simulink model "test_mambo_close_loop"  (R2022b)
settings: Solver=VariableStepAuto  StartTime=0.0  StopTime=20  RelTol=1e-3
values from neighbouring files (symbols this model uses):
  A_angles = sysd_angles.den    [parrot_mambo_main.m]
  Ad = MLD.A    [parrot_mambo_main.m]
  angle_sat = 0.22    [parrot_mambo_main.m]
  B_angles = sysd_angles.num    [parrot_mambo_main.m]
  Bd = MLD.B    [parrot_mambo_main.m]
  Cd = MLD.C    [parrot_mambo_main.m]
  Dd = MLD.D    [parrot_mambo_main.m]
  delay = 0.08    [parrot_mambo_main.m]
  GLOBAL_PARAMETERS = [Ts m g Kv]    [parrot_mambo_main.m]
  K_gain = dlqr(Ad, Bd, Q_gain_lin, R_gain_lin)    [parrot_mambo_main.m]
  K_gain_lin = lqr(A, B, Q_gain_lin, R_gain_lin)    [parrot_mambo_main.m]
  Ts = 0.01    [parrot_mambo_main.m]
settings Model: Creator=phatdo  LastModifiedBy=phatdo

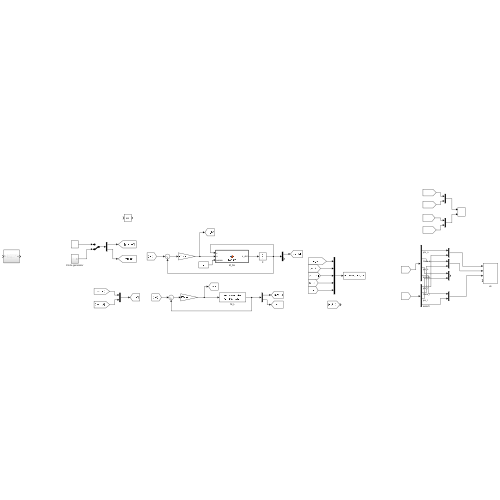
[thumbnail: Simulink's stored preview of the top-level diagram]
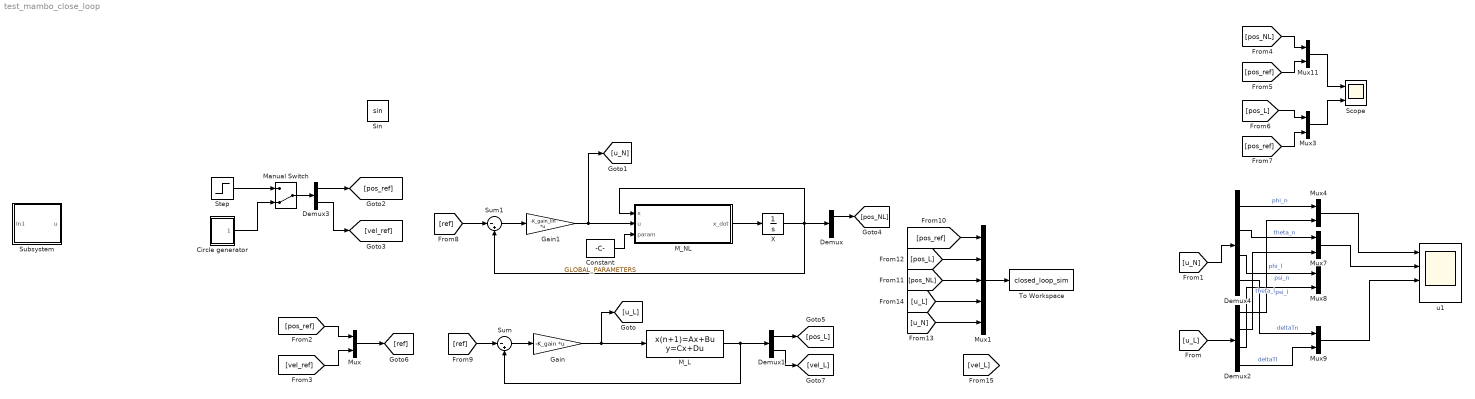
== system test_mambo_close_loop ==
  Circle generator : Subsystem
  Constant : Constant  Value=GLOBAL_PARAMETERS
  Demux : Demux  Outputs=2
  Demux1 : Demux  Outputs=2
  Demux2 : Demux
  Demux3 : Demux  Outputs=2
  Demux4 : Demux
  Gain : Gain  Gain=-K_gain  Multiplication=Matrix(K*u) (u vector)
  Gain1 : Gain  Gain=-K_gain_lin  Multiplication=Matrix(K*u) (u vector)
  M_L : DiscreteStateSpace  A=Ad  B=Bd  C=Cd  D=Dd  SampleTime=-1
  M_NL : MATLAB Function  TreatAsAtomicUnit=on
  Manual Switch : ManualSwitch  CurrentSetting=0
  Mux{,3..4,7..9,11} (7 alike) : Mux  Inputs=2
  Mux1 : Mux  Inputs=5
  Scope : Scope  NumInputPorts=2
  Sin : Trigonometry
  Step : Step  After=[1.5 1.8 2 0 0 0]  SampleTime=Ts
  Subsystem : Subsystem
  Sum : Sum  Inputs=|-+
  Sum1 : Sum  Inputs=|-+
  To Workspace : ToWorkspace  VariableName=closed_loop_sim  SaveFormat=Timeseries  SampleTime=-1
  X : Integrator
  u1 : Scope  NumInputPorts=4
  wires:
  M_L/1 -> Demux1/1, Sum/2
  Sum/1 -> Gain/1
  Gain/1 -> M_L/1, [u_L]
  M_NL/1(x_dot) -> X/1
  Sum1/1 -> Gain1/1
  X/1 -> M_NL/1(x), Demux/1, Sum1/2
  Demux4/1 -> Mux4/1  "phi_n"
  Demux2/1 -> Mux4/2  "phi_l"
  Demux4/2 -> Mux7/1  "theta_n"
  Demux2/2 -> Mux7/2  "theta_l"
  Mux4/1 -> u1/1
  Mux7/1 -> u1/2
  Demux4/3 -> Mux8/1  "psi_n"
  Demux2/3 -> Mux8/2  "psi_l"
  Demux4/4 -> Mux9/1  "deltaTn"
  Demux2/4 -> Mux9/2  "deltaTl"
  Mux9/1 -> u1/3
  Constant/1 -> M_NL/3(param)
  Mux11/1 -> Scope/1
  Gain1/1 -> M_NL/2(u), [u_N]
  [u_L] -> Demux2/1
  [u_N] -> Demux4/1
  Mux3/1 -> Scope/2
  [pos_NL] -> Mux11/1
  [pos_ref] -> Mux11/2
  [pos_L] -> Mux3/1
  [pos_ref] -> Mux3/2
  Demux/1 -> [pos_NL]
  Demux1/1 -> [pos_L]
  [vel_ref] -> Mux/2
  [pos_ref] -> Mux/1
  Mux/1 -> [ref]
  [ref] -> Sum1/1
  [ref] -> Sum/1
  Manual Switch/1 -> Demux3/1
  Circle generator/1(Out1) -> Manual Switch/2
  Demux3/1 -> [pos_ref]
  Demux3/2 -> [vel_ref]
  Step/1 -> Manual Switch/1
  [pos_ref] -> Mux1/1
  Mux1/1 -> To Workspace/1
  [pos_L] -> Mux1/2
  [pos_NL] -> Mux1/3
  [u_L] -> Mux1/4
  [u_N] -> Mux1/5
  Demux1/2 -> [vel_L]

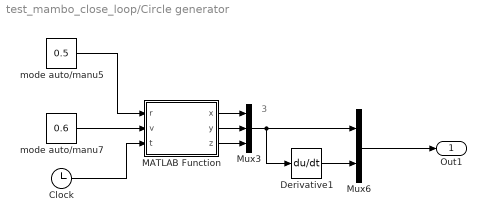
== system test_mambo_close_loop/Circle generator ==
  note: 3
  Clock : Clock
  Derivative1 : Derivative  CoefficientInTFapproximation=4*Ts
  MATLAB Function : MATLAB Function  TreatAsAtomicUnit=on
  Mux3 : Mux  Inputs=3
  Mux6 : Mux  Inputs=2
  mode auto/manu5 : Constant  Value=0.5  OutDataTypeStr=double
  mode auto/manu7 : Constant  Value=0.6  OutDataTypeStr=double
  Out1 : Outport
  wires:
  MATLAB Function/2(y) -> Mux3/2
  Derivative1/1 -> Mux6/2
  Mux3/1 -> Mux6/1, Derivative1/1
  Mux6/1 -> Out1/1
  mode auto/manu5/1 -> MATLAB Function/1(r)
  Clock/1 -> MATLAB Function/3(t)
  MATLAB Function/1(x) -> Mux3/1
  mode auto/manu7/1 -> MATLAB Function/2(v)
  MATLAB Function/3(z) -> Mux3/3

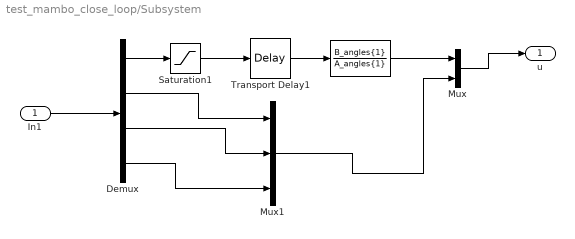
== system test_mambo_close_loop/Subsystem ==
  In1 : Inport
  " " : DiscreteTransferFcn  Numerator=B_angles{1}  Denominator=A_angles{1}  SampleTime=Ts
  Demux : Demux
  Mux : Mux  Inputs=2
  Mux1 : Mux  Inputs=3
  Saturation1 : Saturate  UpperLimit=angle_sat  LowerLimit=-angle_sat
  Transport Delay1 : TransportDelay  DelayTime=delay
  u : Outport
  wires:
  In1/1 -> Demux/1
  Demux/2 -> Mux1/1
  Demux/3 -> Mux1/2
  Transport Delay1/1 -> " "/1
  Saturation1/1 -> Transport Delay1/1
  Demux/1 -> Saturation1/1
  " "/1 -> Mux/1
  Demux/4 -> Mux1/3
  Mux1/1 -> Mux/2
  Mux/1 -> u/1

== matlab function test_mambo_close_loop/M_NL ==
  data: x input; u input; x_dot output; param input
function x_dot = system(x,u, param)
%% Init
% x = [x y z x_dot y_dot z_dot]
% u = [phi theta psi delta_T]

Ts = param(1);
m = param(2);
g = param(3); 
Kv = param(4);

x_dot = zeros(6,1);

%% Output
c_phi   = cos(u(1));
c_theta = cos(u(2));
c_psi   = cos(u(3));
s_phi   = sin(u(1));
s_theta = sin(u(2));
s_psi   = sin(u(3));
deltaT = u(4);

T = deltaT + m*g;

x_dot(1) = x(4);
x_dot(2) = x(5);
x_dot(3) = x(6);
x_dot(4) = (c_phi*s_theta*c_psi + s_phi*s_psi)*T/m;
x_dot(5) = (c_phi*s_theta*s_psi - s_phi*c_psi)*T/m;
x_dot(6) = -g + c_phi*c_theta*T/m;

end

== matlab function test_mambo_close_loop/Circle generator/MATLAB Function ==
  data: x output; r input; y output; v input; t input; z output
function [x,y,z]= fcn(r,v,t)
w=v/r;
x=r*cos(w*t);
y=r*sin(w*t);
z=2;
